simulink model "control_Loop1"  (Simulink 8.1)
settings: Solver=ode45  StartTime=0.0  StopTime=10.0  RelTol=1e-3
settings Model: Creator=wbernal  LastModifiedBy=wbernal
settings DataIOCC: SignalLoggingSaveFormat=Dataset
settings OptimizationCC: ExpressionDepthLimit=128
settings DebuggingCC: FcnCallInpInsideContextMsg=EnableAllAsError
settings GRTTargetCC: CombineOutputUpdateFcns=on  GRTInterface=off

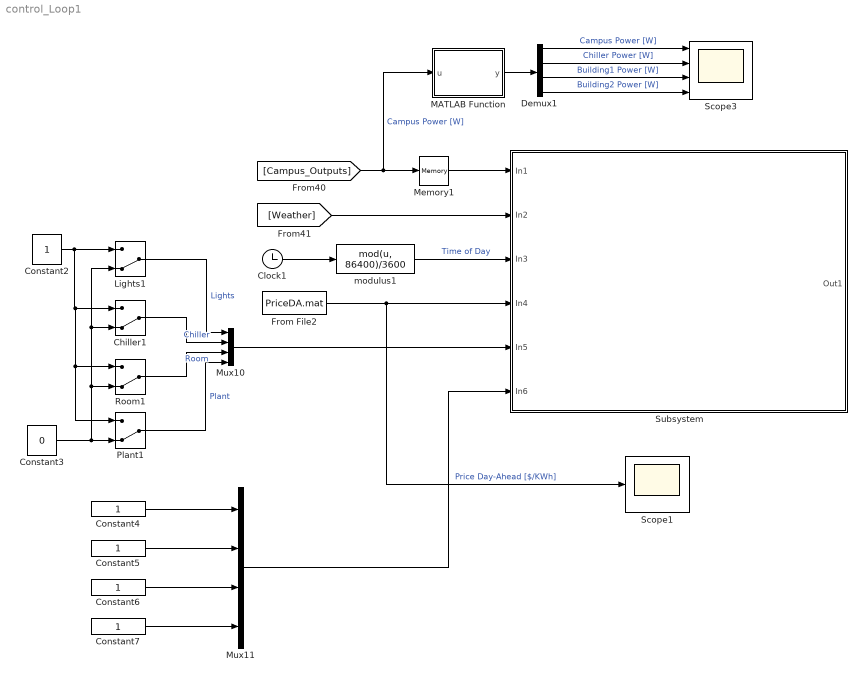
== system control_Loop1 ==
  Chiller1 : ManualSwitch  CurrentSetting=0
  Clock1 : Clock
  Constant{2,4..7} (5 alike) : Constant
  Constant3 : Constant  Value=0
  Demux1 : Demux
  From File2 : FromFile  FileName=PriceDA.mat  SampleTime=0
  Lights1 : ManualSwitch  CurrentSetting=0
  MATLAB Function : MATLAB Function  TreatAsAtomicUnit=on
  Memory1 : Memory
  Mux10 : Mux
  Mux11 : Mux
  Plant1 : ManualSwitch  CurrentSetting=0
  Room1 : ManualSwitch  CurrentSetting=0
  Scope1 : Scope
      settings: TimeRange=86400  YMin=0.0225  YMax=0.06
  Scope3 : Scope  NumInputPorts=4
      settings: TimeRange=86400  YMin=0.0225~-5~-5~-5  YMax=0.06~5~5~5
  Subsystem : Subsystem
  modulus1 : MATLABFcn  MATLABFcn=mod(u, 86400)/3600
  wires:
  [Campus_Outputs] -> MATLAB Function/1(u), Memory1/1  "Campus Power [W]"
  [Weather] -> Subsystem/2(In2)
  Memory1/1 -> Subsystem/1(In1)
  Clock1/1 -> modulus1/1
  modulus1/1 -> Subsystem/3(In3)  "Time of Day"
  From File2/1 -> Scope1/1, Subsystem/4(In4)  "Price Day-Ahead [$/KWh]"
  Mux10/1 -> Subsystem/5(In5)
  Constant2/1 -> Plant1/1, Room1/1, Chiller1/1, Lights1/1
  Chiller1/1 -> Mux10/2  "Chiller"
  Room1/1 -> Mux10/3  "Room"
  Lights1/1 -> Mux10/1  "Lights"
  Plant1/1 -> Mux10/4  "Plant"
  Constant3/1 -> Lights1/2, Chiller1/2, Room1/2, Plant1/2
  MATLAB Function/1(y) -> Demux1/1
  Demux1/1 -> Scope3/1  "Campus Power [W]"
  Demux1/2 -> Scope3/2  "Chiller Power [W]"
  Demux1/4 -> Scope3/4  "Building2 Power [W]"
  Demux1/3 -> Scope3/3  "Building1 Power [W]"
  Mux11/1 -> Subsystem/6(In6)
  Constant4/1 -> Mux11/1
  Constant5/1 -> Mux11/2
  Constant6/1 -> Mux11/3
  Constant7/1 -> Mux11/4

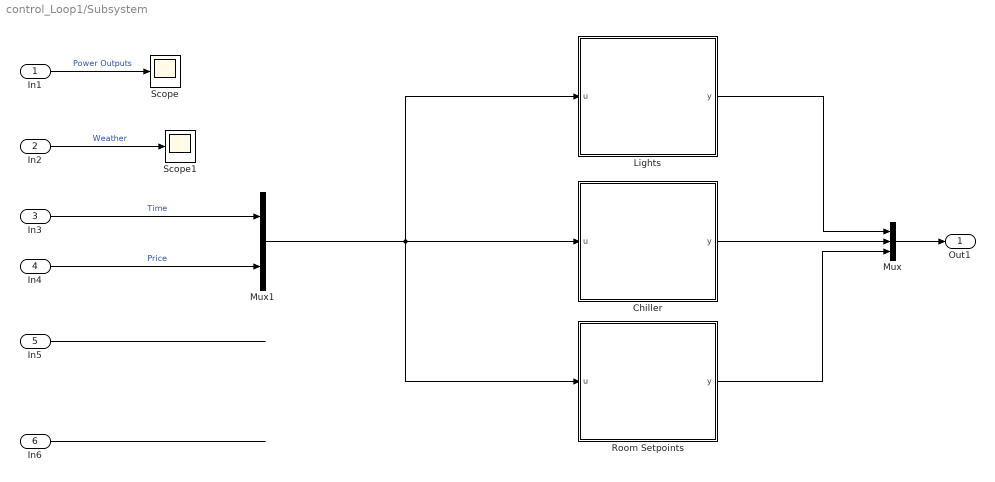
== system control_Loop1/Subsystem ==
  In1 : Inport
  In2 : Inport  Port=2
  In3 : Inport  Port=3
  In4 : Inport  Port=4
  In5 : Inport  Port=5
  In6 : Inport  Port=6
  Chiller : MATLAB Function  TreatAsAtomicUnit=on
  Lights : MATLAB Function  TreatAsAtomicUnit=on
  Mux : Mux  Inputs=3
  Mux1 : Mux  Inputs=2
  Room Setpoints : MATLAB Function  TreatAsAtomicUnit=on
  Scope : Scope
      settings: SaveName=ScopeData12
  Scope1 : Scope
      settings: SaveName=ScopeData13
  Out1 : Outport
  wires:
  In2/1 -> Scope1/1  "Weather"
  In3/1 -> Mux1/1  "Time"
  In5/1 -> ?
  In6/1 -> ?
  Mux/1 -> Out1/1
  Room Setpoints/1(y) -> Mux/3
  Chiller/1(y) -> Mux/2
  Lights/1(y) -> Mux/1
  In1/1 -> Scope/1  "Power Outputs"
  In4/1 -> Mux1/2  "Price"
  Mux1/1 -> Room Setpoints/1(u), Chiller/1(u), Lights/1(u)

== matlab function MATLAB Function ==
  data: u input double; y output double
function y = fcn(u)
%#codegen

y = u;

== matlab function Subsystem/Lights ==
  data: u input double; y output double
function y = fcn(u)
%#codegen

y = u;

== matlab function Subsystem/Chiller ==
  data: u input double; y output double
function y = fcn(u)
%#codegen

y = u;

== matlab function Subsystem/Room Setpoints ==
  data: u input double; y output double
function y = fcn(u)
%#codegen

y = u;
